simulink model "Fourteen_bus"  (R2024a)
settings: Solver=ode23t  StartTime=0.0  StopTime=1  FixedStep=0.2  RelTol=1e-4  AbsTol=1e-6  EnableMultiTasking=on
undefined symbols (not defined in the file): D1, Delta
libraries: neural x24, spsThreePhaseSeriesRLCBranchLib x20, spsThreePhaseVIMeasurementLib x18, spsThreePhaseSeriesRLCLoadLib x11, spsIGBTDiodeLib x6, spsThreePhaseSourceLib x5, spsThreePhaseTransformerTwoWindingsLib x5, spsSeriesRLCBranchLib x4, spsAlphaBetaZerotodq0Lib x2, eePowerMeasurement x2, spsabctodq0Lib x2, slpidlib x1
(part 1 of 2)
settings Model: Creator=Bharath  LastModifiedBy=HP
settings SolverCC: AutoScaleAbsTol=off  MaxConsecutiveMinStep=auto  ZeroCrossControl=DisableAll  AlgebraicLoopSolver=TrustRegion
settings DataIOCC: LimitDataPoints=on  SaveFormat=Array  SignalLoggingSaveFormat=ModelDataLogs  ReturnWorkspaceOutputs=off
settings OptimizationCC: ExpressionDepthLimit=2147483647  LifeSpan=inf
settings DebuggingCC: UnderspecifiedInitializationDetection=Classic  MergeDetectMultiDrivingBlocksExec=none  FcnCallInpInsideContextMsg=warning  UnconnectedInputMsg=warning  UnconnectedOutputMsg=warning  UnconnectedLineMsg=warning  StateNameClashWarn=warning  SFUnexpectedBacktrackingDiag=warning  SFNoUnconditionalDefaultTransitionDiag=warning  SFExecutionAtInitializationDiag=none  ArithmeticOperatorsInVariantConditions=warning
settings HardwareCC: ProdBitPerPointer=32  ProdBitPerSizeT=32  ProdBitPerPtrDiffT=32  ProdLargestAtomicFloat=None  ProdIntDivRoundTo=Undefined  ProdEndianess=Unspecified  ProdWordSize=32  ProdHWDeviceType=32-bit Generic
settings ModelReferenceCC: PropagateSignalLabelsOutOfModel=off
settings SFSimCC: SimUseLocalCustomCode=off  CustomCodeUndefinedFunction=UseInterfaceOnly
settings RTWCC: RTWUseLocalCustomCode=off  GPUComputeCapability=3.5
settings CodeAppCC: StateflowObjectComments=on
settings GRTTargetCC: TargetLangStandard=C89/C90 (ANSI)  CombineOutputUpdateFcns=off  GRTInterface=on
settings ConfigComp: CovMetricSettings=dw  CovSaveCumulativeToWorkspaceVar=on  CovSaveSingleToWorkspaceVar=on  CovExternalEMLEnable=off
settings SimscapeCC: SimscapeNormalizeSystem=off

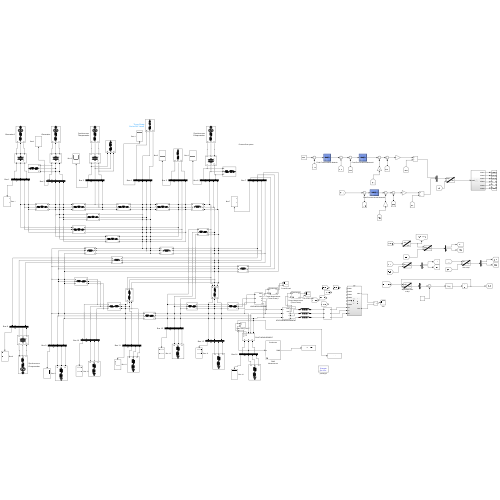
[thumbnail: Simulink's stored preview of the top-level diagram]
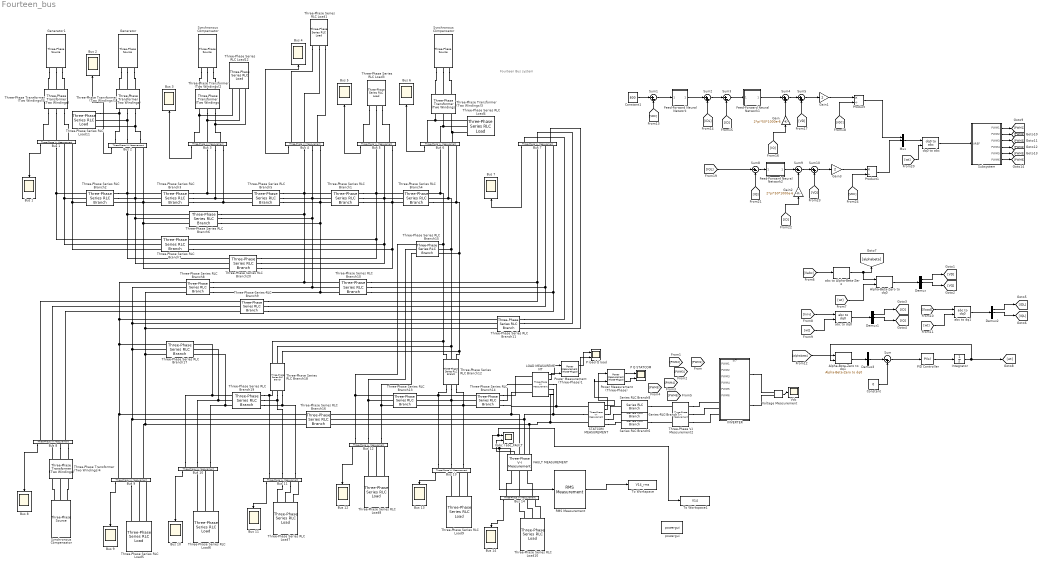
== system Fourteen_bus ==
  note: Fourteen Bus system
  " Generator" : spsThreePhaseSourceLib/Three-Phase Source  InternalConnection=Yg  VoltagePhases=off  Voltage=1.045  PhaseAngle=-30  Voltage_phases=[25e3 25e3 25e3]/sqrt(3)  PhaseAngles_phases=[0 -120 +120]  Frequency=50  NonIdealSource=on  SpecifyImpedance=on  Resistance=0.8929  Inductance=16.58e-3  ShortCircuitLevel=10  BaseVoltage=1  XRratio=1  BusType=PV  Pref=0.4  Qref=0  Prefabc=[10e3, 10e3, 10e3]  Qrefabc=[0, 0, 0]  Qmin=-0.4  Qmax=0.5
  " Generator1" : spsThreePhaseSourceLib/Three-Phase Source  InternalConnection=Yg  VoltagePhases=off  Voltage=1.06  PhaseAngle=-30  Voltage_phases=[25e3 25e3 25e3]/sqrt(3)  PhaseAngles_phases=[0 -120 +120]  Frequency=50  NonIdealSource=on  SpecifyImpedance=on  Resistance=0.8929  Inductance=16.58e-3  ShortCircuitLevel=10  BaseVoltage=1  XRratio=1  BusType=PQ  Pref=2.324  Qref=-0.169  Prefabc=[10e3, 10e3, 10e3]  Qrefabc=[0, 0, 0]  Qmin=0  Qmax=0
  Alpha-Beta-Zero to dq0 : spsAlphaBetaZerotodq0Lib/Alpha-Beta-Zero to dq0  Alignment=90 degrees behind phase A axis
  Alpha-Beta-Zero to dq1 : spsAlphaBetaZerotodq0Lib/Alpha-Beta-Zero to dq0  Alignment=90 degrees behind phase A axis
  Bus {1..14} (14 alike) : Scope
  "Bus 1 " : spsThreePhaseVIMeasurementLib/Three-Phase V-I Measurement  VoltageMeasurement=phase-to-ground  SetLabelV=off  LabelV=Vabc  Vpu=on  VpuLL=off  CurrentMeasurement=yes  SetLabelI=off  LabelI=Iabc  Ipu=on  Pbase=100e6  Vbase=0.95  OutputType=Complex  PhasorSimulation=off  PSBequivalent=0
  "Bus 10 " : spsThreePhaseVIMeasurementLib/Three-Phase V-I Measurement  VoltageMeasurement=phase-to-ground  SetLabelV=off  LabelV=Vabc  Vpu=on  VpuLL=off  CurrentMeasurement=yes  SetLabelI=off  LabelI=Iabc  Ipu=on  Pbase=100e6  Vbase=0.94  OutputType=Complex  PhasorSimulation=off  PSBequivalent=0
  "Bus 11 " : spsThreePhaseVIMeasurementLib/Three-Phase V-I Measurement  VoltageMeasurement=phase-to-ground  SetLabelV=off  LabelV=Vabc  Vpu=on  VpuLL=off  CurrentMeasurement=yes  SetLabelI=off  LabelI=Iabc  Ipu=on  Pbase=100e6  Vbase=0.95  OutputType=Complex  PhasorSimulation=off  PSBequivalent=0
  "Bus 12 " : spsThreePhaseVIMeasurementLib/Three-Phase V-I Measurement  VoltageMeasurement=phase-to-ground  SetLabelV=off  LabelV=Vabc  Vpu=on  VpuLL=off  CurrentMeasurement=yes  SetLabelI=off  LabelI=Iabc  Ipu=on  Pbase=100e6  Vbase=0.95  OutputType=Complex  PhasorSimulation=off  PSBequivalent=0
  "Bus 13 " : spsThreePhaseVIMeasurementLib/Three-Phase V-I Measurement  VoltageMeasurement=phase-to-ground  SetLabelV=off  LabelV=Vabc  Vpu=on  VpuLL=off  CurrentMeasurement=yes  SetLabelI=off  LabelI=Iabc  Ipu=on  Pbase=100e6  Vbase=0.95  OutputType=Complex  PhasorSimulation=off  PSBequivalent=0
  "Bus 14 " : spsThreePhaseVIMeasurementLib/Three-Phase V-I Measurement  VoltageMeasurement=phase-to-ground  SetLabelV=off  LabelV=Vabc  Vpu=on  VpuLL=off  CurrentMeasurement=yes  SetLabelI=off  LabelI=Iabc  Ipu=on  Pbase=100e6  Vbase=0.92  OutputType=Complex  PhasorSimulation=off  PSBequivalent=0
  "Bus 2 " : spsThreePhaseVIMeasurementLib/Three-Phase V-I Measurement  VoltageMeasurement=phase-to-ground  SetLabelV=off  LabelV=Vabc  Vpu=on  VpuLL=off  CurrentMeasurement=yes  SetLabelI=off  LabelI=Iabc  Ipu=on  Pbase=100e6  Vbase=0.95  OutputType=Complex  PhasorSimulation=off  PSBequivalent=0
  "Bus 3 " : spsThreePhaseVIMeasurementLib/Three-Phase V-I Measurement  VoltageMeasurement=phase-to-ground  SetLabelV=off  LabelV=Vabc  Vpu=on  VpuLL=off  CurrentMeasurement=yes  SetLabelI=off  LabelI=Iabc  Ipu=on  Pbase=100e6  Vbase=0.95  OutputType=Complex  PhasorSimulation=off  PSBequivalent=0
  "Bus 4 " : spsThreePhaseVIMeasurementLib/Three-Phase V-I Measurement  VoltageMeasurement=phase-to-ground  SetLabelV=off  LabelV=Vabc  Vpu=on  VpuLL=off  CurrentMeasurement=yes  SetLabelI=off  LabelI=Iabc  Ipu=on  Pbase=100e6  Vbase=0.95  OutputType=Complex  PhasorSimulation=off  PSBequivalent=0
  "Bus 5 " : spsThreePhaseVIMeasurementLib/Three-Phase V-I Measurement  VoltageMeasurement=phase-to-ground  SetLabelV=off  LabelV=Vabc  Vpu=on  VpuLL=off  CurrentMeasurement=yes  SetLabelI=off  LabelI=Iabc  Ipu=on  Pbase=100e6  Vbase=0.95  OutputType=Complex  PhasorSimulation=off  PSBequivalent=0
  "Bus 6 " : spsThreePhaseVIMeasurementLib/Three-Phase V-I Measurement  VoltageMeasurement=phase-to-ground  SetLabelV=off  LabelV=Vabc  Vpu=on  VpuLL=off  CurrentMeasurement=yes  SetLabelI=off  LabelI=Iabc  Ipu=on  Pbase=100e6  Vbase=0.95  OutputType=Complex  PhasorSimulation=off  PSBequivalent=0
  "Bus 7 " : spsThreePhaseVIMeasurementLib/Three-Phase V-I Measurement  VoltageMeasurement=phase-to-ground  SetLabelV=off  LabelV=Vabc  Vpu=on  VpuLL=off  CurrentMeasurement=yes  SetLabelI=off  LabelI=Iabc  Ipu=off  Pbase=100e6  Vbase=0.95  OutputType=Complex  PhasorSimulation=off  PSBequivalent=0
  "Bus 8 " : spsThreePhaseVIMeasurementLib/Three-Phase V-I Measurement  VoltageMeasurement=phase-to-ground  SetLabelV=off  LabelV=Vabc  Vpu=on  VpuLL=off  CurrentMeasurement=yes  SetLabelI=off  LabelI=Iabc  Ipu=on  Pbase=100e6  Vbase=1  OutputType=Complex  PhasorSimulation=off  PSBequivalent=0
  "Bus 9 " : spsThreePhaseVIMeasurementLib/Three-Phase V-I Measurement  VoltageMeasurement=phase-to-ground  SetLabelV=off  LabelV=Vabc  Vpu=on  VpuLL=off  CurrentMeasurement=yes  SetLabelI=off  LabelI=Iabc  Ipu=on  Pbase=100e6  Vbase=0.94  OutputType=Complex  PhasorSimulation=off  PSBequivalent=0
  Constant : Constant  Value=0
  Constant1 : Constant  Value=800
  Demux{,1..3} (4 alike) : Demux  Outputs=3
  FAULT MEASUREMENT : spsThreePhaseVIMeasurementLib/Three-Phase V-I Measurement  VoltageMeasurement=phase-to-ground  SetLabelV=off  LabelV=Vabc  Vpu=off  VpuLL=off  CurrentMeasurement=yes  SetLabelI=off  LabelI=Iabc  Ipu=off  Pbase=100e6  Vbase=500e3  OutputType=Complex  PhasorSimulation=off  PSBequivalent=0
  Feed-Forward Neural Network : Subsystem
      mask help: Feed-Forward Neural Network
      mask Display: e = 0.06;c1 = [120 150 230]/255;c2 = ([120 150 230]+0)/383;c3 = ([120 150 230]+128)/383;patch([0 1 1 0],[0 0 1 1],c1);patch([0 1 1 1-e 1-e 0+e],[0 0 1 1-e 0+e 0+e],c2);patch([0 0 1 1-e 0+e 0+e],[0 1 1 1-e 1-e 0+e],c3);plot([0 1 1 0 0],[0 0 1 1 0]);fprintf('NNET');port_label('input',1,' Input');port_label('output',1,'Output ');
  Feed-Forward Neural Network1 : Subsystem
      mask help: Feed-Forward Neural Network
      mask Display: e = 0.06;c1 = [120 150 230]/255;c2 = ([120 150 230]+0)/383;c3 = ([120 150 230]+128)/383;patch([0 1 1 0],[0 0 1 1],c1);patch([0 1 1 1-e 1-e 0+e],[0 0 1 1-e 0+e 0+e],c2);patch([0 0 1 1-e 0+e 0+e],[0 1 1 1-e 1-e 0+e],c3);plot([0 1 1 0 0],[0 0 1 1 0]);fprintf('NNET');port_label('input',1,' Input');port_label('output',1,'Output ');
  Feed-Forward Neural Network2 : Subsystem
      mask help: Feed-Forward Neural Network
      mask Display: e = 0.06;c1 = [120 150 230]/255;c2 = ([120 150 230]+0)/383;c3 = ([120 150 230]+128)/383;patch([0 1 1 0],[0 0 1 1],c1);patch([0 1 1 1-e 1-e 0+e],[0 0 1 1-e 0+e 0+e],c2);patch([0 0 1 1-e 0+e 0+e],[0 1 1 1-e 1-e 0+e],c3);plot([0 1 1 0 0],[0 0 1 1 0]);fprintf('NNET');port_label('input',1,' Input');port_label('output',1,'Output ');
  Gain : Gain  Gain=2*pi*50*1000e-6
  Gain1 : Gain  Gain=2
  Gain2 : Gain  Gain=2*pi*50*1000e-6
  Gain3 : Gain  Gain=2
  INVERTER : Subsystem
      settings: PortSchema="{\"entries\":[{\"content\":{\"sides\":[{\"content\":{\"connectorIds\":[\"In1\",\"In2\",\"In3\",\"In4\",\"In5\",\"In6\",\"LConn1\",\"LConn2\",\"LConn3\"]},\"type\":\"ConnectorPlacement.EquallySpacedRectSide\",\"uuid\":\"cd926914-e500-44bb-a824-1c24039a7a05\"},{\"content\":{\"connectorIds\":[\"RConn1\",\"RConn2\"],\"side\":\"RIGHT\"},\"type\":\"ConnectorPlacement.EquallySpacedRectSide\",\"uuid\":\"b5fe95d9-c13f-4751-8149-0110a2c0a406\"},{\"content\":{\"connectorIds\":[\"In7\"],\"side\":\"TOP\"},\"type\":\"ConnectorPlacement.EquallySpacedRectSide\",\"uuid\":\"79979526-b8a1-4432-a367-ea42808a9205\"}]},\"type\":\"ConnectorPlacement.EquallySpacedConnector\",\"uuid\":\"d4d72b20-a28b-42a9-a273-2f88ea46e899\"}],\"packageUris\":[\"http://schema.mathworks.com/mf0/Connector/R2020b\"],\"version\":\"1.0\"}"
  Integrator : Integrator
  LOAD MEASUREMENT : spsThreePhaseVIMeasurementLib/Three-Phase V-I Measurement  VoltageMeasurement=phase-to-ground  SetLabelV=off  LabelV=Vabc  Vpu=off  VpuLL=off  CurrentMeasurement=yes  SetLabelI=off  LabelI=Iabc  Ipu=off  Pbase=100e6  Vbase=500e3  OutputType=Complex  PhasorSimulation=off  PSBequivalent=0
  Mux : Mux  Inputs=3
  P Q STATCOM : Scope  NumInputPorts=2
  P load Q load : Scope  NumInputPorts=2
  PID Controller : slpidlib/PID Controller  Controller=PI  Form=Parallel  TimeDomain=Continuous-time  UseExternalTs=off  SampleTime=-1  IntegratorMethod=Forward Euler  FilterMethod=Forward Euler  ControllerParametersSource=internal  P=10  I=50000  UseKiTs=off  D=0  UseExternalDerivativeSource=off  N=100  UseFilter=on  TunerSelectOption=Transfer Function Based (PID Tuner App)  InitialConditionSource=internal  InitialConditionForIntegrator=0  InitialConditionForFilter=0  DifferentiatorICPrevScaledInput=0  ExternalReset=none  TrackingMode=off  Kt=1  LimitOutput=off  SatLimitsSource=internal  UpperSaturationLimit=inf  LowerSaturationLimit=-inf  LinearizeAsGain=on  AntiWindupMode=none  Kb=1  LimitIntegrator=off  UpperIntegratorSaturationLimit=inf  LowerIntegratorSaturationLimit=-inf  POutMin=[]  POutMax=[]  IOutMin=[]  IOutMax=[]  DOutMin=[]  DOutMax=[]  NOutMin=[]  NOutMax=[]  SumOutMin=[]  SumOutMax=[]  SaturationOutMin=[]  SaturationOutMax=[]  PParamMin=[]  PParamMax=[]  IParamMin=[]  IParamMax=[]  DParamMin=[]  DParamMax=[]  NParamMin=[]  NParamMax=[]  KbParamMin=[]  KbParamMax=[]  KtParamMin=[]  KtParamMax=[]  KbOutMin=[]  KbOutMax=[]  KtOutMin=[]  KtOutMax=[]  IntegratorOutMin=[]  IntegratorOutMax=[]  FilterOutMin=[]  FilterOutMax=[]  SumI1OutMin=[]  SumI1OutMax=[]  SumI2OutMin=[]  SumI2OutMax=[]  SumI3OutMin=[]  SumI3OutMax=[]  SumI4OutMin=[]  SumI4OutMax=[]  SumDOutMin=[]  SumDOutMax=[]  DifferentiatorOutMin=[]  DifferentiatorOutMax=[]  FilterDiffOutCoefMin=[]  FilterDiffOutCoefMax=[]  ReciprocalOutMin=[]  ReciprocalOutMax=[]  SumDenOutMin=[]  SumDenOutMax=[]  SumNumOutMin=[]  SumNumOutMax=[]  DivideOutMin=[]  DivideOutMax=[]  UdiffTsProdOutMin=[]  UdiffTsProdOutMax=[]  NTsProdOutMin=[]  NTsProdOutMax=[]  UintegralTsProdOutMin=[]  UintegralTsProdOutMax=[]  UngainTsProdOutMin=[]  UngainTsProdOutMax=[]  ClampingZeroOutDataTypeStr=Inherit: Inherit via back propagation  ClampingZeroOutMin=[]  ClampingZeroOutMax=[]  FilterDenConstantOutDataTypeStr=Inherit: Inherit via back propagation  FilterDenConstantOutMin=[]  FilterDenConstantOutMax=[]  PCopyOutDataTypeStr=Inherit: Inherit via back propagation  PCopyOutMin=[]  PCopyOutMax=[]  NCopyOutDataTypeStr=Inherit: Inherit via back propagation  NCopyOutMin=[]  NCopyOutMax=[]  IntegratorContinuousStateAttributes=''  IntegratorStateMustResolveToSignalObject=off  IntegratorRTWStateStorageClass=Auto  FilterContinuousStateAttributes=''  FilterStateMustResolveToSignalObject=off  FilterRTWStateStorageClass=Auto  ParallelPVariant=InternalParameters  IdealPVariant=Disabled  IVariant=InternalParameters  DVariant=Disabled  IntegratorVariant=Continuous  SatVariant=Disabled  AWVariant=Passthrough  PCopyVariant=Disabled  TRVariant=Disabled  FdbkBlocksVariant=Forward  IdealPFdbkVariant=Disabled  SatFdbkVariant=Disabled  DerivativeFilterVariant=Disabled  NVariant=Disabled  NCopyVariant=Disabled_SignalSpec  FilterICVariant=Disabled  IntegratorICVariant=InternalICs  ExternalResetVariant=Disabled  TRSumVariant=Passthrough  SumFdbkVariant=Disabled  SumVariant=Sum_PI  TsampFilterVariant=InternalTs  TsampNgainVariant=Passthrough  TsampIntegralVariant=Disabled_SignalSpec  ExternalSaturationOutDataTypeStr=Inherit: Same as second input  DerivativeSourceVariant=Disabled
  Power Measurement (Three-Phase) : eePowerMeasurement/Power Measurement (Three-Phase)  LabelModeActiveChoice=Continuous  F=60  K=[0 1 2 3]  Seq=Positive  Ts=0
  Power Measurement (Three-Phase)1 : eePowerMeasurement/Power Measurement (Three-Phase)  LabelModeActiveChoice=Continuous  F=60  K=[0 1 2 3]  Seq=Positive  Ts=0
  Product : Product  Inputs=*/
  Product1 : Product  Inputs=*/
  RMS Measurement : eeRmsMeasurement/RMS Measurement  LabelModeActiveChoice=Total  F=50  SpecifyHarmonics=off  K=[1]  Ts=0
      settings: LibrarySourceBlock=|
      | ee_sl_lib/Measurements/RMS
      | Measurement
  STATCOM MEASUREMENT : spsThreePhaseVIMeasurementLib/Three-Phase V-I Measurement  VoltageMeasurement=phase-to-ground  SetLabelV=off  LabelV=Vabc  Vpu=off  VpuLL=off  CurrentMeasurement=yes  SetLabelI=off  LabelI=Iabc  Ipu=off  Pbase=100e6  Vbase=500e3  OutputType=Complex  PhasorSimulation=off  PSBequivalent=0
  Series RLC Branch6 : spsSeriesRLCBranchLib/Series RLC Branch  LConnTagsString=__new0  RConnTagsString=__new0  BranchType=L  Resistance=1  Inductance=500e-6  SetiL0=off  InitialCurrent=0  Capacitance=1e-6  Setx0=off  InitialVoltage=0  Measurements=None
  Series RLC Branch7 : spsSeriesRLCBranchLib/Series RLC Branch  LConnTagsString=__new0  RConnTagsString=__new0  BranchType=L  Resistance=1  Inductance=500e-6  SetiL0=off  InitialCurrent=0  Capacitance=1e-6  Setx0=off  InitialVoltage=0  Measurements=None
  Series RLC Branch8 : spsSeriesRLCBranchLib/Series RLC Branch  LConnTagsString=__new0  RConnTagsString=__new0  BranchType=L  Resistance=1  Inductance=500e-6  SetiL0=off  InitialCurrent=0  Capacitance=1e-6  Setx0=off  InitialVoltage=0  Measurements=None
  Subsystem : Subsystem
  Sum : Sum  Inputs=|-+
  Sum{1,3,8..9} (4 alike) : Sum  Inputs=|+-
  Sum{2,4..5,10} (4 alike) : Sum  Inputs=|++
  Synchronous Compensator : spsThreePhaseSourceLib/Three-Phase Source  InternalConnection=Yg  VoltagePhases=off  Voltage=1.09  PhaseAngle=-30  Voltage_phases=[25e3 25e3 25e3]/sqrt(3)  PhaseAngles_phases=[0 -120 +120]  Frequency=50  NonIdealSource=on  SpecifyImpedance=on  Resistance=0.8929  Inductance=16.58e-3  ShortCircuitLevel=10  BaseVoltage=1  XRratio=1  BusType=PV  Pref=0  Qref=0  Prefabc=[10e3, 10e3, 10e3]  Qrefabc=[0, 0, 0]  Qmin=-0.06  Qmax=0.24
  Synchronous Compensator : spsThreePhaseSourceLib/Three-Phase Source  InternalConnection=Yg  VoltagePhases=off  Voltage=1.01  PhaseAngle=-30  Voltage_phases=[25e3 25e3 25e3]/sqrt(3)  PhaseAngles_phases=[0 -120 +120]  Frequency=50  NonIdealSource=on  SpecifyImpedance=on  Resistance=0.8929  Inductance=16.58e-3  ShortCircuitLevel=10  BaseVoltage=1  XRratio=1  BusType=PV  Pref=0  Qref=23.4e6  Prefabc=[10e3, 10e3, 10e3]  Qrefabc=[0, 0, 0]  Qmin=0  Qmax=0.4
  "Synchronous Compensator " : spsThreePhaseSourceLib/Three-Phase Source  InternalConnection=Yg  VoltagePhases=off  Voltage=1.07  PhaseAngle=-30  Voltage_phases=[25e3 25e3 25e3]/sqrt(3)  PhaseAngles_phases=[0 -120 +120]  Frequency=50  NonIdealSource=on  SpecifyImpedance=on  Resistance=0.8929  Inductance=16.58e-3  ShortCircuitLevel=10  BaseVoltage=1  XRratio=1  BusType=PV  Pref=0  Qref=23.4e6  Prefabc=[10e3, 10e3, 10e3]  Qrefabc=[0, 0, 0]  Qmin=-0.06  Qmax=0.24
  Three-Phase Series RLC Branch1 : spsThreePhaseSeriesRLCBranchLib/Three-Phase Series RLC Branch  LConnTagsString=A|B|C  RConnTagsString=A|B|C  BranchType=RLC  Resistance=0.01335  Inductance=0.04211/(2*pi*50)  Capacitance=1/0.0128/(2*pi*50)  Measurements=None
  Three-Phase Series RLC Branch10 : spsThreePhaseSeriesRLCBranchLib/Three-Phase Series RLC Branch  LConnTagsString=A|B|C  RConnTagsString=A|B|C  BranchType=L  Resistance=1  Inductance=0.20912/(2*pi*50)  Capacitance=1e-6  Measurements=None
  Three-Phase Series RLC Branch11 : spsThreePhaseSeriesRLCBranchLib/Three-Phase Series RLC Branch  LConnTagsString=A|B|C  RConnTagsString=A|B|C  BranchType=L  Resistance=1  Inductance=0.11001/(2*pi*50)  Capacitance=1e-6  Measurements=None
  Three-Phase Series RLC Branch12 : spsThreePhaseSeriesRLCBranchLib/Three-Phase Series RLC Branch  LConnTagsString=A|B|C  RConnTagsString=A|B|C  BranchType=RL  Resistance=0.06615  Inductance=0.13027/(2*pi*50)  Capacitance=1e-6  Measurements=None
  Three-Phase Series RLC Branch13 : spsThreePhaseSeriesRLCBranchLib/Three-Phase Series RLC Branch  LConnTagsString=A|B|C  RConnTagsString=A|B|C  BranchType=RL  Resistance=0.22092  Inductance=0.19988/(2*pi*50)  Capacitance=1e-6  Measurements=None
  Three-Phase Series RLC Branch14 : spsThreePhaseSeriesRLCBranchLib/Three-Phase Series RLC Branch  LConnTagsString=A|B|C  RConnTagsString=A|B|C  BranchType=RL  Resistance=0.17093  Inductance=0.34802/(2*pi*50)  Capacitance=1e-6  Measurements=None
  Three-Phase Series RLC Branch15 : spsThreePhaseSeriesRLCBranchLib/Three-Phase Series RLC Branch  LConnTagsString=A|B|C  RConnTagsString=A|B|C  BranchType=RL  Resistance=0.12291  Inductance=0.25581/(2*pi*50)  Capacitance=1e-6  Measurements=None
  Three-Phase Series RLC Branch16 : spsThreePhaseSeriesRLCBranchLib/Three-Phase Series RLC Branch  LConnTagsString=A|B|C  RConnTagsString=A|B|C  BranchType=RL  Resistance=0.12711  Inductance=0.27038/(2*pi*50)  Capacitance=1e-6  Measurements=None
  Three-Phase Series RLC Branch17 : spsThreePhaseSeriesRLCBranchLib/Three-Phase Series RLC Branch  LConnTagsString=A|B|C  RConnTagsString=A|B|C  BranchType=RL  Resistance=0.03181  Inductance=0.08450/(2*pi*50)  Capacitance=1e-6  Measurements=None
  Three-Phase Series RLC Branch18 : spsThreePhaseSeriesRLCBranchLib/Three-Phase Series RLC Branch  LConnTagsString=A|B|C  RConnTagsString=A|B|C  BranchType=RL  Resistance=0.09498  Inductance=0.1989/(2*pi*50)  Capacitance=1e-6  Measurements=None
  Three-Phase Series RLC Branch19 : spsThreePhaseSeriesRLCBranchLib/Three-Phase Series RLC Branch  LConnTagsString=A|B|C  RConnTagsString=A|B|C  BranchType=RL  Resistance=0.08205  Inductance=0.19207/(2*pi*50)  Capacitance=1e-6  Measurements=None
  Three-Phase Series RLC Branch2 : spsThreePhaseSeriesRLCBranchLib/Three-Phase Series RLC Branch  LConnTagsString=A|B|C  RConnTagsString=A|B|C  BranchType=RLC  Resistance=0.01938  Inductance=0.05917/(2*pi*50)  Capacitance=1/0.0528/(2*pi*50)  Measurements=None
  Three-Phase Series RLC Branch20 : spsThreePhaseSeriesRLCBranchLib/Three-Phase Series RLC Branch  LConnTagsString=A|B|C  RConnTagsString=A|B|C  BranchType=RLC  Resistance=0.05695  Inductance=0.17388/(2*pi*50)  Capacitance=1/0.0340/(2*pi*50)  Measurements=None
  Three-Phase Series RLC Branch3 : spsThreePhaseSeriesRLCBranchLib/Three-Phase Series RLC Branch  LConnTagsString=A|B|C  RConnTagsString=A|B|C  BranchType=RLC  Resistance=0.04699  Inductance=0.19797/(2*pi*50)  Capacitance=1/0.0438/(2*pi*50)  Measurements=None
  Three-Phase Series RLC Branch4 : spsThreePhaseSeriesRLCBranchLib/Three-Phase Series RLC Branch  LConnTagsString=A|B|C  RConnTagsString=A|B|C  BranchType=L  Resistance=1  Inductance=0.25202/(2*pi*50)  Capacitance=1e-6  Measurements=None
  Three-Phase Series RLC Branch5 : spsThreePhaseSeriesRLCBranchLib/Three-Phase Series RLC Branch  LConnTagsString=A|B|C  RConnTagsString=A|B|C  BranchType=RLC  Resistance=0.06701  Inductance=0.17103/(2*pi*50)  Capacitance=1/0.0346/(2*pi*50)  Measurements=None
  Three-Phase Series RLC Branch6 : spsThreePhaseSeriesRLCBranchLib/Three-Phase Series RLC Branch  LConnTagsString=A|B|C  RConnTagsString=A|B|C  BranchType=RLC  Resistance=0.05811  Inductance=0.17632/(2*pi*50)  Capacitance=1/0.0374/(2*pi*50)  Measurements=None
  Three-Phase Series RLC Branch7 : spsThreePhaseSeriesRLCBranchLib/Three-Phase Series RLC Branch  LConnTagsString=A|B|C  RConnTagsString=A|B|C  BranchType=RLC  Resistance=0.05403  Inductance=0.22304/(2*pi*50)  Capacitance=1/0.0492/(2*pi*50)  Measurements=None
  Three-Phase Series RLC Branch8 : spsThreePhaseSeriesRLCBranchLib/Three-Phase Series RLC Branch  LConnTagsString=A|B|C  RConnTagsString=A|B|C  BranchType=L  Resistance=1  Inductance=0.55618/(2*pi*50)  Capacitance=1e-6  Measurements=None
  Three-Phase Series RLC Branch9 : spsThreePhaseSeriesRLCBranchLib/Three-Phase Series RLC Branch  LConnTagsString=A|B|C  RConnTagsString=A|B|C  BranchType=L  Resistance=1  Inductance=0.17615/(2*pi*50)  Capacitance=1e-6  Measurements=None
  Three-Phase Series RLC Load1 : spsThreePhaseSeriesRLCLoadLib/Three-Phase Series RLC Load  LConnTagsString=A|B|C  Configuration=Y (grounded)  NominalVoltage=1  Vabc=[1e3 1e3 1e3]  Vabcp=[1e3 1e3 1e3]  NominalFrequency=50  UnbalancedPower=off  ActivePower=0.478  InductivePower=0  CapacitivePower=0.039  Pabc=[10e3 9e3 11e3]  QLabc=[100 90 110]  QCabc=[100 90 110]  Pabcp=[10e3 9e3 11e3]  QLabcp=[100 90 110]  QCabcp=[100 90 110]  Measurements=None  LoadType=constant PQ
  Three-Phase Series RLC Load10 : spsThreePhaseSeriesRLCLoadLib/Three-Phase Series RLC Load  LConnTagsString=A|B|C  Configuration=Y (grounded)  NominalVoltage=1  Vabc=[1e3 1e3 1e3]  Vabcp=[1e3 1e3 1e3]  NominalFrequency=50  UnbalancedPower=off  ActivePower=0.149  InductivePower=0.050  CapacitivePower=0  Pabc=[10e3 9e3 11e3]  QLabc=[100 90 110]  QCabc=[100 90 110]  Pabcp=[10e3 9e3 11e3]  QLabcp=[100 90 110]  QCabcp=[100 90 110]  Measurements=None  LoadType=constant Z
  Three-Phase Series RLC Load11 : spsThreePhaseSeriesRLCLoadLib/Three-Phase Series RLC Load  LConnTagsString=A|B|C  Configuration=Y (grounded)  NominalVoltage=1  Vabc=[1e3 1e3 1e3]  Vabcp=[1e3 1e3 1e3]  NominalFrequency=50  UnbalancedPower=off  ActivePower=0.217  InductivePower=0.127  CapacitivePower=0  Pabc=[10e3 9e3 11e3]  QLabc=[100 90 110]  QCabc=[100 90 110]  Pabcp=[10e3 9e3 11e3]  QLabcp=[100 90 110]  QCabcp=[100 90 110]  Measurements=None  LoadType=constant PQ
  Three-Phase Series RLC Load12 : spsThreePhaseSeriesRLCLoadLib/Three-Phase Series RLC Load  LConnTagsString=A|B|C  Configuration=Y (grounded)  NominalVoltage=1  Vabc=[1e3 1e3 1e3]  Vabcp=[1e3 1e3 1e3]  NominalFrequency=50  UnbalancedPower=off  ActivePower=0.942  InductivePower=0.191  CapacitivePower=0  Pabc=[10e3 9e3 11e3]  QLabc=[100 90 110]  QCabc=[100 90 110]  Pabcp=[10e3 9e3 11e3]  QLabcp=[100 90 110]  QCabcp=[100 90 110]  Measurements=None  LoadType=constant PQ
  Three-Phase Series RLC Load3 : spsThreePhaseSeriesRLCLoadLib/Three-Phase Series RLC Load  LConnTagsString=A|B|C  Configuration=Y (grounded)  NominalVoltage=1  Vabc=[1e3 1e3 1e3]  Vabcp=[1e3 1e3 1e3]  NominalFrequency=50  UnbalancedPower=off  ActivePower=0.076  InductivePower=0.016  CapacitivePower=0  Pabc=[10e3 9e3 11e3]  QLabc=[100 90 110]  QCabc=[100 90 110]  Pabcp=[10e3 9e3 11e3]  QLabcp=[100 90 110]  QCabcp=[100 90 110]  Measurements=None  LoadType=constant PQ
  Three-Phase Series RLC Load4 : spsThreePhaseSeriesRLCLoadLib/Three-Phase Series RLC Load  LConnTagsString=A|B|C  Configuration=Y (grounded)  NominalVoltage=1  Vabc=[1e3 1e3 1e3]  Vabcp=[1e3 1e3 1e3]  NominalFrequency=50  UnbalancedPower=off  ActivePower=0.112  InductivePower=0.075  CapacitivePower=0  Pabc=[10e3 9e3 11e3]  QLabc=[100 90 110]  QCabc=[100 90 110]  Pabcp=[10e3 9e3 11e3]  QLabcp=[100 90 110]  QCabcp=[100 90 110]  Measurements=None  LoadType=constant PQ
  Three-Phase Series RLC Load5 : spsThreePhaseSeriesRLCLoadLib/Three-Phase Series RLC Load  LConnTagsString=A|B|C  Configuration=Y (grounded)  NominalVoltage=1  Vabc=[1e3 1e3 1e3]  Vabcp=[1e3 1e3 1e3]  NominalFrequency=50  UnbalancedPower=off  ActivePower=0.295  InductivePower=0.166  CapacitivePower=0  Pabc=[10e3 9e3 11e3]  QLabc=[100 90 110]  QCabc=[100 90 110]  Pabcp=[10e3 9e3 11e3]  QLabcp=[100 90 110]  QCabcp=[100 90 110]  Measurements=None  LoadType=constant PQ
  Three-Phase Series RLC Load6 : spsThreePhaseSeriesRLCLoadLib/Three-Phase Series RLC Load  LConnTagsString=A|B|C  Configuration=Y (grounded)  NominalVoltage=1  Vabc=[1e3 1e3 1e3]  Vabcp=[1e3 1e3 1e3]  NominalFrequency=50  UnbalancedPower=off  ActivePower=0.09  InductivePower=0.058  CapacitivePower=0  Pabc=[10e3 9e3 11e3]  QLabc=[100 90 110]  QCabc=[100 90 110]  Pabcp=[10e3 9e3 11e3]  QLabcp=[100 90 110]  QCabcp=[100 90 110]  Measurements=None  LoadType=constant PQ
  Three-Phase Series RLC Load7 : spsThreePhaseSeriesRLCLoadLib/Three-Phase Series RLC Load  LConnTagsString=A|B|C  Configuration=Y (grounded)  NominalVoltage=1  Vabc=[1e3 1e3 1e3]  Vabcp=[1e3 1e3 1e3]  NominalFrequency=50  UnbalancedPower=off  ActivePower=0.035  InductivePower=0.018  CapacitivePower=0  Pabc=[10e3 9e3 11e3]  QLabc=[100 90 110]  QCabc=[100 90 110]  Pabcp=[10e3 9e3 11e3]  QLabcp=[100 90 110]  QCabcp=[100 90 110]  Measurements=None  LoadType=constant PQ
  Three-Phase Series RLC Load8 : spsThreePhaseSeriesRLCLoadLib/Three-Phase Series RLC Load  LConnTagsString=A|B|C  Configuration=Y (grounded)  NominalVoltage=1  Vabc=[1e3 1e3 1e3]  Vabcp=[1e3 1e3 1e3]  NominalFrequency=50  UnbalancedPower=off  ActivePower=0.061  InductivePower=0.016  CapacitivePower=0  Pabc=[10e3 9e3 11e3]  QLabc=[100 90 110]  QCabc=[100 90 110]  Pabcp=[10e3 9e3 11e3]  QLabcp=[100 90 110]  QCabcp=[100 90 110]  Measurements=None  LoadType=constant PQ
  Three-Phase Series RLC Load9 : spsThreePhaseSeriesRLCLoadLib/Three-Phase Series RLC Load  LConnTagsString=A|B|C  Configuration=Y (grounded)  NominalVoltage=1  Vabc=[1e3 1e3 1e3]  Vabcp=[1e3 1e3 1e3]  NominalFrequency=50  UnbalancedPower=off  ActivePower=0.135  InductivePower=0.058  CapacitivePower=0  Pabc=[10e3 9e3 11e3]  QLabc=[100 90 110]  QCabc=[100 90 110]  Pabcp=[10e3 9e3 11e3]  QLabcp=[100 90 110]  QCabcp=[100 90 110]  Measurements=None  LoadType=constant PQ
  Three-Phase Transformer (Two Windings)1 : spsThreePhaseTransformerTwoWindingsLib/Three-Phase Transformer (Two Windings)  Winding1Connection=Delta (D1)  Winding2Connection=Yg  CoreType=Three single-phase transformers  SetSaturation=off  Hysteresis=off  DataFile='hysteresis'  SetInitialFlux=off  Measurements=None  UNITS=pu  NominalPower=[ 1 , 50 ]  Winding1=[ 1.045 , 0.002 , 0.08 ]  Winding2=[ 1.045 , 0.002 , 0.08 ]  Rm=500  Lm=500  L0=0.5  Saturation=[ 0,0 ; 0.0024,1.2 ; 1.0,1.52 ]  InitialFluxes=[ 0.8 , -0.8 , 0.7 ]  BreakLoop=off  DiscreteSolver=Trapezoidal iterative  DataType=off  TransfoNumber=1
  Three-Phase Transformer (Two Windings)2 : spsThreePhaseTransformerTwoWindingsLib/Three-Phase Transformer (Two Windings)  Winding1Connection=Delta (D1)  Winding2Connection=Yg  CoreType=Three single-phase transformers  SetSaturation=off  Hysteresis=off  DataFile='hysteresis'  SetInitialFlux=off  Measurements=None  UNITS=pu  NominalPower=[ 1 , 50 ]  Winding1=[ 1.01 , 0.002 , 0.08 ]  Winding2=[ 1.01 , 0.002 , 0.08 ]  Rm=500  Lm=500  L0=0.5  Saturation=[ 0,0 ; 0.0024,1.2 ; 1.0,1.52 ]  InitialFluxes=[ 0.8 , -0.8 , 0.7 ]  BreakLoop=off  DiscreteSolver=Trapezoidal iterative  DataType=off  TransfoNumber=1
  Three-Phase Transformer (Two Windings)3 : spsThreePhaseTransformerTwoWindingsLib/Three-Phase Transformer (Two Windings)  Winding1Connection=Delta (D1)  Winding2Connection=Yg  CoreType=Three single-phase transformers  SetSaturation=off  Hysteresis=off  DataFile='hysteresis'  SetInitialFlux=off  Measurements=None  UNITS=pu  NominalPower=[ 1 , 50 ]  Winding1=[ 1.07 , 0.002 , 0.08 ]  Winding2=[ 1.07 , 0.002 , 0.08 ]  Rm=500  Lm=500  L0=0.5  Saturation=[ 0,0 ; 0.0024,1.2 ; 1.0,1.52 ]  InitialFluxes=[ 0.8 , -0.8 , 0.7 ]  BreakLoop=off  DiscreteSolver=Trapezoidal iterative  DataType=off  TransfoNumber=1
  Three-Phase Transformer (Two Windings)4 : spsThreePhaseTransformerTwoWindingsLib/Three-Phase Transformer (Two Windings)  Winding1Connection=Yg  Winding2Connection=Delta (D1)  CoreType=Three single-phase transformers  SetSaturation=off  Hysteresis=off  DataFile='hysteresis'  SetInitialFlux=off  Measurements=None  UNITS=pu  NominalPower=[ 1 , 50 ]  Winding1=[ 1.09 , 0.002 , 0.08]  Winding2=[1.09 , 0.002 , 0.08]  Rm=500  Lm=500  L0=0.5  Saturation=[0 0;0.0023999 1.2;1 1.52]  InitialFluxes=[0.80002 -0.80002 0.69999]  BreakLoop=off  DiscreteSolver=Trapezoidal iterative  DataType=off  TransfoNumber=1
  Three-Phase Transformer (Two Windings)5 : spsThreePhaseTransformerTwoWindingsLib/Three-Phase Transformer (Two Windings)  Winding1Connection=Delta (D1)  Winding2Connection=Yg  CoreType=Three single-phase transformers  SetSaturation=off  Hysteresis=off  DataFile='hysteresis'  SetInitialFlux=off  Measurements=None  UNITS=pu  NominalPower=[ 1 , 50 ]  Winding1=[ 1.06 , 0.002 , 0.08 ]  Winding2=[ 1.06 , 0.002 , 0.08 ]  Rm=500  Lm=500  L0=0.5  Saturation=[ 0,0 ; 0.0024,1.2 ; 1.0,1.52 ]  InitialFluxes=[ 0.8 , -0.8 , 0.7 ]  BreakLoop=off  DiscreteSolver=Trapezoidal iterative  DataType=off  TransfoNumber=1
  Three-Phase V-I Measurement2 : spsThreePhaseVIMeasurementLib/Three-Phase V-I Measurement  VoltageMeasurement=phase-to-ground  SetLabelV=on  LabelV=Vinv  Vpu=off  VpuLL=off  CurrentMeasurement=yes  SetLabelI=on  LabelI=Iinv  Ipu=off  Pbase=100e6  Vbase=500e3  OutputType=Complex  PhasorSimulation=off  PSBequivalent=0
  To Workspace : ToWorkspace  VariableName=V14_rms  SampleTime=-1
  To Workspace1 : ToWorkspace  VariableName=V14  SaveFormat=Structure With Time  SampleTime=-1
  Vabc I abc_FAULT : Scope  NumInputPorts=2
  Vdc : Scope
  Voltage Measurement : spsVoltageMeasurementLib/Voltage Measurement  PhasorSimulation=off  OutputType=Complex  PSBequivalent=0
  abc to Alpha-Beta-Zero : spsabctoAlphaBetaZeroLib/abc to Alpha-Beta-Zero
  abc to dq0 : spsabctodq0Lib/abc to dq0  Alignment=90 degrees behind phase A axis
  abc to dq1 : spsabctodq0Lib/abc to dq0  Alignment=90 degrees behind phase A axis
  dq0 to abc : spsdq0toabcLib/dq0 to abc  Alignment=90 degrees behind phase A axis
  powergui : spspowerguiLib/powergui  Priority=1  SimulationMode=Discrete  SampleTime=50e-6  frequency=60  Iterations=50  frequencyindice=0  Pbase=100e6  ErrMax=1e-4  UnitsV=kV  UnitsW=MW  buscounter=0  FunctionMessages=off  echomessages=off  EnableUseOfTLC=off  CurrentSourceSwitches=on  DisableSnubberDevices=off  DisableRonSwitches=off  DisableVfSwitches=off  DisplayEquations=off  AutomaticDiscreteSolvers=off  SolverType=Tustin  Interpol=off  ExternalGateDelay=off  methode=off  Ts=100  x0status=blocks  SPID=off  SwTol=0  HookPort=off  NonlinearTolerance=1e-4  nMaxIteration=100  ContinueOnMaxIteration=off  RestoreLinks=warning  ResistiveCurrentMeasurement=off  Frange=[0:2:500]  Ylog=off  Xlog=on  ShowGrid=off  save=off  variable=ZData  structure=0  ZoomFFT=off  StartTime=0.0  cycles=1  DisplayStyle=1  fundamental=60  FreqAxis=off  MaxFrequency=1000  frequencyindicesteady=1  RmsSteady=1  display=off
  wires:
  "Bus 11 "/1 -> Bus 11/1
  "Bus 10 "/1 -> Bus 10/1
  "Bus 9 "/1 -> Bus 9/1
  "Bus 8 "/1 -> Bus 8/1
  "Bus 7 "/1 -> Bus 7/1
  "Bus 4 "/1 -> Bus 4/1
  "Bus 2 "/1 -> Bus 2/1
  "Bus 14 "/1 -> Bus 14/1
  "Bus 13 "/1 -> Bus 13/1
  "Bus 12 "/1 -> Bus 12/1
  "Bus 5 "/1 -> Bus 5/1
  "Bus 1 "/1 -> Bus 1/1
  "Bus 3 "/1 -> Bus 3/1
  "Bus 6 "/1 -> Bus 6/1
  Subsystem/5(PWM5) -> [PWM5]
  [IQ] -> Gain/1
  [VDC] -> Product/2
  Constant1/1 -> Sum1/1
  Feed-Forward Neural Network1/1(Output) -> Sum4/1
  Sum4/1 -> Sum5/1
  [ID] -> Gain2/1
  Product1/1 -> Mux/2
  [VDC] -> Sum1/2
  [VD] -> Sum5/2
  Subsystem/2(PWM2) -> [PWM2]
  dq0 to abc/1 -> Subsystem/1(VREF)
  Feed-Forward Neural Network/1(Output) -> Sum2/1
  Sum10/1 -> Gain3/1
  Gain1/1 -> Product/1
  Subsystem/3(PWM3) -> [PWM3]
  [VDC] -> Product1/2
  Subsystem/1(PWM1) -> [PWM1]
  [VQ] -> Sum10/2
  Sum5/1 -> Gain1/1
  [ID] -> Sum3/2
  Product/1 -> Mux/1
  Sum2/1 -> Sum3/1
  Gain/1 -> Sum4/2
  Gain3/1 -> Product1/1
  Subsystem/4(PWM4) -> [PWM4]
  Sum9/1 -> Sum10/1
  Mux/1 -> dq0 to abc/1
  Sum8/1 -> Feed-Forward Neural Network2/1(Input)
  [wt] -> dq0 to abc/2
  Gain2/1 -> Sum9/2
  Feed-Forward Neural Network2/1(Output) -> Sum9/1
  [IDL] -> Sum2/2
  Sum3/1 -> Feed-Forward Neural Network1/1(Input)
  [IQL] -> Sum8/1
  Subsystem/6(PWM6) -> [PWM6]
  [IQ] -> Sum8/2
  Sum1/1 -> Feed-Forward Neural Network/1(Input)
  PID Controller/1 -> Integrator/1
  Demux2/2 -> [IQL]
  Constant/1 -> Sum/2
  Demux1/2 -> [IQ]
  abc to dq1/1 -> Demux2/1
  [Vabc] -> abc to Alpha-Beta-Zero/1
  [Iload] -> abc to dq1/1
  Demux3/2 -> Sum/1
  Alpha-Beta-Zero to dq1/1 -> Demux3/1
  abc to dq0/1 -> Demux1/1
  Demux2/1 -> [IDL]
  Demux/1 -> [VD]
  abc to Alpha-Beta-Zero/1 -> [alphabeta], Alpha-Beta-Zero to dq0/1
  [wt] -> Alpha-Beta-Zero to dq0/2
  [wt] -> abc to dq0/2
  [wt] -> abc to dq1/2
  Alpha-Beta-Zero to dq0/1 -> Demux/1
  Sum/1 -> PID Controller/1
  Demux1/1 -> [ID]
  Demux/2 -> [VQ]
  [alphabeta] -> Alpha-Beta-Zero to dq1/1
  [Iinv] -> abc to dq0/1
  Integrator/1 -> Alpha-Beta-Zero to dq1/2, [wt]
  Voltage Measurement/1 -> Vdc/1
  FAULT MEASUREMENT/1 -> RMS Measurement/1, To Workspace1/1, Vabc I abc_FAULT/1
  FAULT MEASUREMENT/2 -> Vabc I abc_FAULT/2
  STATCOM MEASUREMENT/1 -> Power Measurement (Three-Phase)/1
  STATCOM MEASUREMENT/2 -> Power Measurement (Three-Phase)/2
  Power Measurement (Three-Phase)/1 -> P Q STATCOM/1
  Power Measurement (Three-Phase)/2 -> P Q STATCOM/2
  LOAD MEASUREMENT/1 -> Power Measurement (Three-Phase)1/1
  LOAD MEASUREMENT/2 -> Power Measurement (Three-Phase)1/2
  Power Measurement (Three-Phase)1/1 -> P load Q load/1
  Power Measurement (Three-Phase)1/2 -> P load Q load/2
  RMS Measurement/1 -> To Workspace/1
  connections:
  Three-Phase Series RLC Branch16/RConn3 -- "Bus 9 "/LConn3 -- Three-Phase Series RLC Branch17/RConn3 -- Three-Phase Series RLC Branch11/RConn3 -- Three-Phase Series RLC Branch8/LConn3
  Three-Phase Series RLC Branch16/RConn2 -- "Bus 9 "/LConn2 -- Three-Phase Series RLC Branch17/RConn2 -- Three-Phase Series RLC Branch11/RConn2 -- Three-Phase Series RLC Branch8/LConn2
  Three-Phase Series RLC Branch16/RConn1 -- "Bus 9 "/LConn1 -- Three-Phase Series RLC Branch17/RConn1 -- Three-Phase Series RLC Branch11/RConn1 -- Three-Phase Series RLC Branch8/LConn1
  "Bus 7 "/RConn3 -- Three-Phase Series RLC Branch10/RConn3 -- Three-Phase Series RLC Branch9/RConn3
  "Bus 7 "/RConn2 -- Three-Phase Series RLC Branch10/RConn2 -- Three-Phase Series RLC Branch9/RConn2
  "Bus 7 "/RConn1 -- Three-Phase Series RLC Branch10/RConn1 -- Three-Phase Series RLC Branch9/RConn1
  "Bus 6 "/RConn3 -- Three-Phase Series RLC Branch12/LConn3 -- Three-Phase Series RLC Branch18/LConn3 -- Three-Phase Series RLC Branch15/LConn3 -- Three-Phase Series RLC Branch4/RConn3
  "Bus 6 "/RConn2 -- Three-Phase Series RLC Branch15/LConn2 -- Three-Phase Series RLC Branch18/LConn2 -- Three-Phase Series RLC Branch12/LConn2 -- Three-Phase Series RLC Branch4/RConn2
  "Bus 6 "/RConn1 -- Three-Phase Series RLC Branch18/LConn1 -- Three-Phase Series RLC Branch12/LConn1 -- Three-Phase Series RLC Branch15/LConn1 -- Three-Phase Series RLC Branch4/RConn1
  "Bus 5 "/RConn3 -- Three-Phase Series RLC Branch1/RConn3 -- Three-Phase Series RLC Branch20/RConn3 -- Three-Phase Series RLC Branch7/RConn3 -- Three-Phase Series RLC Branch4/LConn3
  "Bus 5 "/RConn2 -- Three-Phase Series RLC Branch1/RConn2 -- Three-Phase Series RLC Branch20/RConn2 -- Three-Phase Series RLC Branch7/RConn2 -- Three-Phase Series RLC Branch4/LConn2
  "Bus 5 "/RConn1 -- Three-Phase Series RLC Branch1/RConn1 -- Three-Phase Series RLC Branch20/RConn1 -- Three-Phase Series RLC Branch7/RConn1 -- Three-Phase Series RLC Branch4/LConn1
  "Bus 3 "/RConn2 -- Three-Phase Series RLC Branch5/LConn2 -- Three-Phase Series RLC Branch3/RConn2
  "Bus 3 "/RConn1 -- Three-Phase Series RLC Branch5/LConn1 -- Three-Phase Series RLC Branch3/RConn1
  "Bus 2 "/RConn3 -- Three-Phase Series RLC Branch20/LConn3 -- Three-Phase Series RLC Branch6/LConn3 -- Three-Phase Series RLC Branch3/LConn3 -- Three-Phase Series RLC Branch2/RConn3
  "Bus 2 "/RConn2 -- Three-Phase Series RLC Branch20/LConn2 -- Three-Phase Series RLC Branch6/LConn2 -- Three-Phase Series RLC Branch2/RConn2 -- Three-Phase Series RLC Branch3/LConn2
  "Bus 2 "/RConn1 -- Three-Phase Series RLC Branch20/LConn1 -- Three-Phase Series RLC Branch6/LConn1 -- Three-Phase Series RLC Branch2/RConn1 -- Three-Phase Series RLC Branch3/LConn1
  "Bus 2 "/LConn2 -- Three-Phase Series RLC Load11/LConn2 -- Three-Phase Transformer (Two Windings)1/RConn2
  "Bus 2 "/LConn1 -- Three-Phase Series RLC Load11/LConn1 -- Three-Phase Transformer (Two Windings)1/RConn1
  STATCOM MEASUREMENT/LConn3 -- LOAD MEASUREMENT/RConn3 -- FAULT MEASUREMENT/RConn3 -- Three-Phase Series RLC Branch16/LConn3
  STATCOM MEASUREMENT/LConn2 -- LOAD MEASUREMENT/RConn2 -- FAULT MEASUREMENT/RConn2 -- Three-Phase Series RLC Branch16/LConn2
  STATCOM MEASUREMENT/LConn1 -- LOAD MEASUREMENT/RConn1 -- FAULT MEASUREMENT/RConn1 -- Three-Phase Series RLC Branch16/LConn1
  "Bus 13 "/LConn3 -- Three-Phase Series RLC Branch14/RConn3 -- Three-Phase Series RLC Branch12/RConn3 -- Three-Phase Series RLC Branch13/LConn3
  "Bus 13 "/LConn2 -- Three-Phase Series RLC Branch14/RConn2 -- Three-Phase Series RLC Branch12/RConn2 -- Three-Phase Series RLC Branch13/LConn2
  "Bus 13 "/LConn1 -- Three-Phase Series RLC Branch14/RConn1 -- Three-Phase Series RLC Branch12/RConn1 -- Three-Phase Series RLC Branch13/LConn1
  "Bus 12 "/LConn3 -- Three-Phase Series RLC Branch13/RConn3 -- Three-Phase Series RLC Branch15/RConn3
  "Bus 12 "/LConn2 -- Three-Phase Series RLC Branch13/RConn2 -- Three-Phase Series RLC Branch15/RConn2
  "Bus 12 "/LConn1 -- Three-Phase Series RLC Branch13/RConn1 -- Three-Phase Series RLC Branch15/RConn1
  "Bus 11 "/LConn3 -- Three-Phase Series RLC Branch19/RConn3 -- Three-Phase Series RLC Branch18/RConn3
  "Bus 11 "/LConn2 -- Three-Phase Series RLC Branch19/RConn2 -- Three-Phase Series RLC Branch18/RConn2
  "Bus 11 "/LConn1 -- Three-Phase Series RLC Branch19/RConn1 -- Three-Phase Series RLC Branch18/RConn1
  "Bus 10 "/LConn3 -- Three-Phase Series RLC Branch17/LConn3 -- Three-Phase Series RLC Branch19/LConn3
  "Bus 10 "/LConn2 -- Three-Phase Series RLC Branch17/LConn2 -- Three-Phase Series RLC Branch19/LConn2
  "Bus 10 "/LConn1 -- Three-Phase Series RLC Branch19/LConn1 -- Three-Phase Series RLC Branch17/LConn1
  "Bus 1 "/RConn3 -- Three-Phase Series RLC Branch2/LConn3 -- Three-Phase Series RLC Branch7/LConn3
  "Bus 1 "/RConn2 -- Three-Phase Series RLC Branch2/LConn2 -- Three-Phase Series RLC Branch7/LConn2
  "Bus 1 "/RConn1 -- Three-Phase Series RLC Branch2/LConn1 -- Three-Phase Series RLC Branch7/LConn1
  Three-Phase Series RLC Load1/LConn3 -- "Bus 4 "/LConn3
  "Bus 8 "/RConn3 -- Three-Phase Transformer (Two Windings)4/LConn3
  "Bus 8 "/RConn2 -- Three-Phase Transformer (Two Windings)4/LConn2
  Three-Phase Transformer (Two Windings)4/LConn1 -- "Bus 8 "/RConn1
  Three-Phase Series RLC Load5/LConn2 -- "Bus 9 "/RConn2
  "Bus 9 "/RConn1 -- Three-Phase Series RLC Load5/LConn1
  Three-Phase Series RLC Load5/LConn3 -- "Bus 9 "/RConn3
  " Generator"/RConn2 -- Three-Phase Transformer (Two Windings)1/LConn2
  Three-Phase Series RLC Load1/LConn2 -- "Bus 4 "/LConn2
  Three-Phase Series RLC Load3/LConn1 -- "Bus 5 "/LConn1
  Three-Phase Series RLC Load3/LConn3 -- "Bus 5 "/LConn3
  "Bus 7 "/LConn3 -- Three-Phase Series RLC Branch11/LConn3
  Three-Phase Series RLC Load3/LConn2 -- "Bus 5 "/LConn2
  Three-Phase Series RLC Load10/LConn3 -- "Bus 14 "/RConn3
  Three-Phase Series RLC Load10/LConn2 -- "Bus 14 "/RConn2
  Three-Phase Series RLC Load10/LConn1 -- "Bus 14 "/RConn1
  Three-Phase Series RLC Load9/LConn3 -- "Bus 13 "/RConn3
  Three-Phase Series RLC Load9/LConn2 -- "Bus 13 "/RConn2
  Three-Phase Series RLC Load9/LConn1 -- "Bus 13 "/RConn1
  Three-Phase Series RLC Load8/LConn3 -- "Bus 12 "/RConn3
  Three-Phase Series RLC Load8/LConn2 -- "Bus 12 "/RConn2
  Three-Phase Series RLC Load8/LConn1 -- "Bus 12 "/RConn1
  Three-Phase Series RLC Load7/LConn3 -- "Bus 11 "/RConn3
  "Bus 11 "/RConn2 -- Three-Phase Series RLC Load7/LConn2
  "Bus 11 "/RConn1 -- Three-Phase Series RLC Load7/LConn1
  Three-Phase Series RLC Load6/LConn3 -- "Bus 10 "/RConn3
  Three-Phase Series RLC Load6/LConn2 -- "Bus 10 "/RConn2
  Three-Phase Series RLC Load6/LConn1 -- "Bus 10 "/RConn1
  "Bus 2 "/LConn3 -- Three-Phase Series RLC Load11/LConn3 -- Three-Phase Transformer (Two Windings)1/RConn3
  Three-Phase Series RLC Branch9/LConn1 -- "Bus 8 "/LConn1
  Three-Phase Series RLC Branch9/LConn2 -- "Bus 8 "/LConn2
  Three-Phase Series RLC Branch9/LConn3 -- "Bus 8 "/LConn3
  Three-Phase Series RLC Load1/LConn1 -- "Bus 4 "/LConn1
  Three-Phase Series RLC Branch11/LConn2 -- "Bus 7 "/LConn2
  Three-Phase Series RLC Branch11/LConn1 -- "Bus 7 "/LConn1
  Three-Phase Transformer (Two Windings)5/RConn2 -- "Bus 1 "/LConn2
  Three-Phase Transformer (Two Windings)5/RConn1 -- "Bus 1 "/LConn1
  " Generator1"/RConn2 -- Three-Phase Transformer (Two Windings)5/LConn2
  Three-Phase Transformer (Two Windings)5/RConn3 -- "Bus 1 "/LConn3
  Three-Phase Series RLC Load12/LConn2 -- Three-Phase Transformer (Two Windings)2/RConn2 -- "Bus 3 "/LConn2
  Three-Phase Series RLC Load12/LConn1 -- Three-Phase Transformer (Two Windings)2/RConn1 -- "Bus 3 "/LConn1
  Synchronous Compensator/RConn2 -- Three-Phase Transformer (Two Windings)2/LConn2
  Three-Phase Series RLC Load12/LConn3 -- Three-Phase Transformer (Two Windings)2/RConn3 -- "Bus 3 "/LConn3
  "Bus 6 "/LConn2 -- Three-Phase Transformer (Two Windings)3/RConn2 -- Three-Phase Series RLC Load4/LConn2
  "Bus 6 "/LConn1 -- Three-Phase Transformer (Two Windings)3/RConn1 -- Three-Phase Series RLC Load4/LConn1
  "Bus 6 "/LConn3 -- Three-Phase Transformer (Two Windings)3/RConn3 -- Three-Phase Series RLC Load4/LConn3
  "Synchronous Compensator "/RConn2 -- Three-Phase Transformer (Two Windings)3/LConn2
  "Bus 4 "/RConn3 -- Three-Phase Series RLC Branch1/LConn3 -- Three-Phase Series RLC Branch5/RConn3 -- Three-Phase Series RLC Branch6/RConn3 -- Three-Phase Series RLC Branch10/LConn3 -- Three-Phase Series RLC Branch8/RConn3
  "Bus 4 "/RConn2 -- Three-Phase Series RLC Branch5/RConn2 -- Three-Phase Series RLC Branch1/LConn2 -- Three-Phase Series RLC Branch6/RConn2 -- Three-Phase Series RLC Branch10/LConn2 -- Three-Phase Series RLC Branch8/RConn2
  "Bus 4 "/RConn1 -- Three-Phase Series RLC Branch1/LConn1 -- Three-Phase Series RLC Branch6/RConn1 -- Three-Phase Series RLC Branch10/LConn1 -- Three-Phase Series RLC Branch8/RConn1 -- Three-Phase Series RLC Branch5/RConn1
  Synchronous Compensator/RConn2 -- Three-Phase Transformer (Two Windings)4/RConn2
  Synchronous Compensator/RConn3 -- Three-Phase Transformer (Two Windings)4/RConn3
  Synchronous Compensator/RConn1 -- Three-Phase Transformer (Two Windings)4/RConn1
  "Synchronous Compensator "/RConn1 -- Three-Phase Transformer (Two Windings)3/LConn1
  "Synchronous Compensator "/RConn3 -- Three-Phase Transformer (Two Windings)3/LConn3
  " Generator1"/RConn3 -- Three-Phase Transformer (Two Windings)5/LConn3
  " Generator1"/RConn1 -- Three-Phase Transformer (Two Windings)5/LConn1
  Synchronous Compensator/RConn3 -- Three-Phase Transformer (Two Windings)2/LConn3
  Synchronous Compensator/RConn1 -- Three-Phase Transformer (Two Windings)2/LConn1
  " Generator"/RConn1 -- Three-Phase Transformer (Two Windings)1/LConn1
  " Generator"/RConn3 -- Three-Phase Transformer (Two Windings)1/LConn3
  "Bus 3 "/RConn3 -- Three-Phase Series RLC Branch5/LConn3 -- Three-Phase Series RLC Branch3/RConn3
  Three-Phase V-I Measurement2/LConn2 -- INVERTER/LConn2
  Series RLC Branch6/RConn1 -- Three-Phase V-I Measurement2/RConn3
  INVERTER/RConn2 -- Voltage Measurement/LConn2
  Series RLC Branch8/RConn1 -- Three-Phase V-I Measurement2/RConn1
  Three-Phase V-I Measurement2/LConn1 -- INVERTER/LConn1
  Series RLC Branch7/RConn1 -- Three-Phase V-I Measurement2/RConn2
  INVERTER/RConn1 -- Voltage Measurement/LConn1
  Three-Phase V-I Measurement2/LConn3 -- INVERTER/LConn3
  "Bus 14 "/LConn1 -- FAULT MEASUREMENT/LConn1
  "Bus 14 "/LConn2 -- FAULT MEASUREMENT/LConn2
  "Bus 14 "/LConn3 -- FAULT MEASUREMENT/LConn3
  STATCOM MEASUREMENT/RConn1 -- Series RLC Branch8/LConn1
  STATCOM MEASUREMENT/RConn2 -- Series RLC Branch7/LConn1
  STATCOM MEASUREMENT/RConn3 -- Series RLC Branch6/LConn1
  Three-Phase Series RLC Branch14/LConn1 -- LOAD MEASUREMENT/LConn1
  Three-Phase Series RLC Branch14/LConn2 -- LOAD MEASUREMENT/LConn2
  Three-Phase Series RLC Branch14/LConn3 -- LOAD MEASUREMENT/LConn3

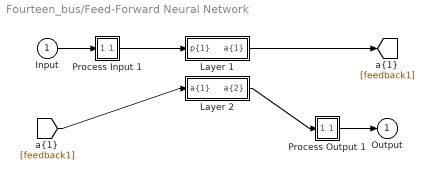
== system Fourteen_bus/Feed-Forward Neural Network ==
  Input : Inport  PortDimensions=1
      mask Display: e = 0.06;c1 = [120 230 180]/255;c2 = ([120 230 180]+0)/(256+128);c3 = ([120 230 180]+128)/(256+128);patch([0 1 1 0],[0 0 1 1],c1);patch([0 1 1 1-e 1-e 0+e],[0 0 1 1-e 0+e 0+e],c2);patch([0 0 1 1-e 0+e 0+e],[0 1 1 1-e 1-e 0+e],c3);plot([0 1 1 0 0],[0 0 1 1 0]);
  Layer 1 : Subsystem
      mask Display: e = 0.06;c1 = [120 150 230]/255;c2 = ([120 150 230]+0)/383;c3 = ([120 150 230]+128)/383;patch([0 1 1 0],[0 0 1 1],c1);patch([0 1 1 1-e 1-e 0+e],[0 0 1 1-e 0+e 0+e],c2);patch([0 0 1 1-e 0+e 0+e],[0 1 1 1-e 1-e 0+e],c3);plot([0 1 1 0 0],[0 0 1 1 0]);
  Layer 2 : Subsystem
      mask Display: e = 0.06;c1 = [120 150 230]/255;c2 = ([120 150 230]+0)/383;c3 = ([120 150 230]+128)/383;patch([0 1 1 0],[0 0 1 1],c1);patch([0 1 1 1-e 1-e 0+e],[0 0 1 1-e 0+e 0+e],c2);patch([0 0 1 1-e 0+e 0+e],[0 1 1 1-e 1-e 0+e],c3);plot([0 1 1 0 0],[0 0 1 1 0]);
  Process Input 1 : Subsystem
      mask Display: e = 0.06;c1 = [120 150 230]/255;c2 = ([120 150 230]+0)/383;c3 = ([120 150 230]+128)/383;patch([0 1 1 0],[0 0 1 1],c1);patch([0 1 1 1-e 1-e 0+e],[0 0 1 1-e 0+e 0+e],c2);patch([0 0 1 1-e 0+e 0+e],[0 1 1 1-e 1-e 0+e],c3);plot([0 1 1 0 0],[0 0 1 1 0]);
  Process Output 1 : Subsystem
      mask Display: e = 0.06;c1 = [120 150 230]/255;c2 = ([120 150 230]+0)/383;c3 = ([120 150 230]+128)/383;patch([0 1 1 0],[0 0 1 1],c1);patch([0 1 1 1-e 1-e 0+e],[0 0 1 1-e 0+e 0+e],c2);patch([0 0 1 1-e 0+e 0+e],[0 1 1 1-e 1-e 0+e],c3);plot([0 1 1 0 0],[0 0 1 1 0]);
  Output : Outport  InitialOutput=0
      mask Display: e = 0.06;c1 = [120 230 180]/255;c2 = ([120 230 180]+0)/(256+128);c3 = ([120 230 180]+128)/(256+128);patch([0 1 1 0],[0 0 1 1],c1);patch([0 1 1 1-e 1-e 0+e],[0 0 1 1-e 0+e 0+e],c2);patch([0 0 1 1-e 0+e 0+e],[0 1 1 1-e 1-e 0+e],c3);plot([0 1 1 0 0],[0 0 1 1 0]);
  wires:
  Input/1 -> Process Input 1/1(x)
  Process Output 1/1(y) -> Output/1
  Process Input 1/1(p) -> Layer 1/1("p{1}")
  Layer 1/1("a{1}") -> [feedback1]
  [feedback1] -> Layer 2/1("a{1} ")
  Layer 2/1("a{2}") -> Process Output 1/1(a)

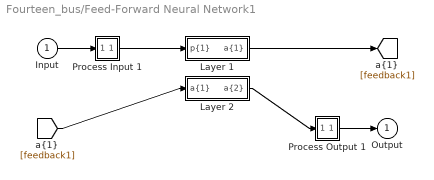
== system Fourteen_bus/Feed-Forward Neural Network1 ==
  Input : Inport  PortDimensions=1
      mask Display: e = 0.06;c1 = [120 230 180]/255;c2 = ([120 230 180]+0)/(256+128);c3 = ([120 230 180]+128)/(256+128);patch([0 1 1 0],[0 0 1 1],c1);patch([0 1 1 1-e 1-e 0+e],[0 0 1 1-e 0+e 0+e],c2);patch([0 0 1 1-e 0+e 0+e],[0 1 1 1-e 1-e 0+e],c3);plot([0 1 1 0 0],[0 0 1 1 0]);
  Layer 1 : Subsystem
      mask Display: e = 0.06;c1 = [120 150 230]/255;c2 = ([120 150 230]+0)/383;c3 = ([120 150 230]+128)/383;patch([0 1 1 0],[0 0 1 1],c1);patch([0 1 1 1-e 1-e 0+e],[0 0 1 1-e 0+e 0+e],c2);patch([0 0 1 1-e 0+e 0+e],[0 1 1 1-e 1-e 0+e],c3);plot([0 1 1 0 0],[0 0 1 1 0]);
  Layer 2 : Subsystem
      mask Display: e = 0.06;c1 = [120 150 230]/255;c2 = ([120 150 230]+0)/383;c3 = ([120 150 230]+128)/383;patch([0 1 1 0],[0 0 1 1],c1);patch([0 1 1 1-e 1-e 0+e],[0 0 1 1-e 0+e 0+e],c2);patch([0 0 1 1-e 0+e 0+e],[0 1 1 1-e 1-e 0+e],c3);plot([0 1 1 0 0],[0 0 1 1 0]);
  Process Input 1 : Subsystem
      mask Display: e = 0.06;c1 = [120 150 230]/255;c2 = ([120 150 230]+0)/383;c3 = ([120 150 230]+128)/383;patch([0 1 1 0],[0 0 1 1],c1);patch([0 1 1 1-e 1-e 0+e],[0 0 1 1-e 0+e 0+e],c2);patch([0 0 1 1-e 0+e 0+e],[0 1 1 1-e 1-e 0+e],c3);plot([0 1 1 0 0],[0 0 1 1 0]);
  Process Output 1 : Subsystem
      mask Display: e = 0.06;c1 = [120 150 230]/255;c2 = ([120 150 230]+0)/383;c3 = ([120 150 230]+128)/383;patch([0 1 1 0],[0 0 1 1],c1);patch([0 1 1 1-e 1-e 0+e],[0 0 1 1-e 0+e 0+e],c2);patch([0 0 1 1-e 0+e 0+e],[0 1 1 1-e 1-e 0+e],c3);plot([0 1 1 0 0],[0 0 1 1 0]);
  Output : Outport  InitialOutput=0
      mask Display: e = 0.06;c1 = [120 230 180]/255;c2 = ([120 230 180]+0)/(256+128);c3 = ([120 230 180]+128)/(256+128);patch([0 1 1 0],[0 0 1 1],c1);patch([0 1 1 1-e 1-e 0+e],[0 0 1 1-e 0+e 0+e],c2);patch([0 0 1 1-e 0+e 0+e],[0 1 1 1-e 1-e 0+e],c3);plot([0 1 1 0 0],[0 0 1 1 0]);
  wires:
  Input/1 -> Process Input 1/1(x)
  Process Output 1/1(y) -> Output/1
  Process Input 1/1(p) -> Layer 1/1("p{1}")
  Layer 1/1("a{1}") -> [feedback1]
  [feedback1] -> Layer 2/1("a{1} ")
  Layer 2/1("a{2}") -> Process Output 1/1(a)
